simulink model "continue_ladrc"  (R2019a)
settings: Solver=VariableStepAuto  StartTime=0.0  StopTime=10.0  RelTol=1e-3
undefined symbols (not defined in the file or in its folder): b0, w0, wc
settings Model: Creator=smilingfrog  LastModifiedBy=smilingfrog

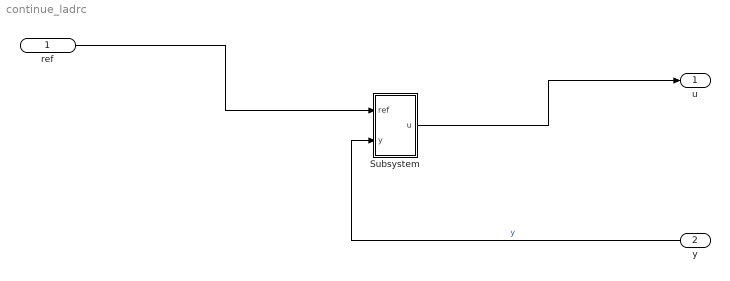
== system continue_ladrc ==
  ref : Inport
  y : Inport  Port=2
  Subsystem : Subsystem
  u : Outport
  wires:
  ref/1 -> Subsystem/1(ref)
  y/1 -> Subsystem/2(y)  "y"
  Subsystem/1(u) -> u/1

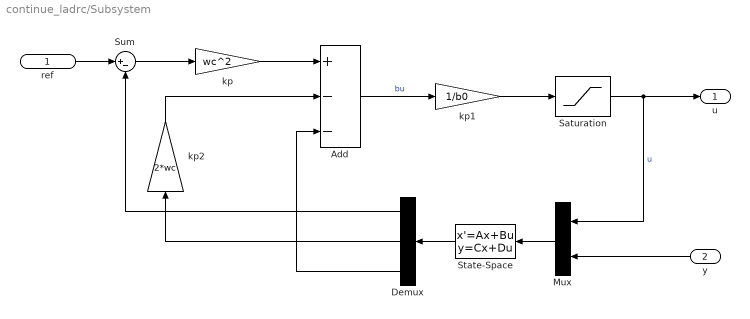
== system continue_ladrc/Subsystem ==
  ref : Inport
  y : Inport  Port=2
  Add : Sum  Inputs=+--
  Demux : Demux  Outputs=3
  Mux : Mux  Inputs=2
  Saturation : Saturate  UpperLimit=0.95  LowerLimit=0.01
  State-Space : StateSpace  A=[-3*w0 1 0;-3*w0^2 0 1;-w0^3 0 0]  B=[0 3*w0;b0 3*w0^2;0 w0^3]  C=[1 0 0;0 1 0;0 0 1]  D=[0 0;0 0;0 0]  InitialCondition=0
  Sum : Sum  Inputs=|+-
  kp : Gain  Gain=wc^2
  kp1 : Gain  Gain=1/b0
  kp2 : Gain  Gain=2*wc
  u : Outport
  wires:
  State-Space/1 -> Demux/1
  Mux/1 -> State-Space/1
  kp/1 -> Add/1
  Demux/1 -> Sum/2
  Saturation/1 -> u/1, Mux/1  "u"
  y/1 -> Mux/2
  ref/1 -> Sum/1
  kp1/1 -> Saturation/1
  Sum/1 -> kp/1
  Demux/2 -> kp2/1
  Demux/3 -> Add/3
  Add/1 -> kp1/1  "bu"
  kp2/1 -> Add/2
